simulink model "ANS_GFM_short_term"  (R2021b)
settings: Solver=FixedStepAuto  StartTime=0.0  StopTime=5  FixedStep=Ts  MaxStep=1e-5  RelTol=1e-3
values from neighbouring files (symbols this model uses):
  angle_load = angle(LF.bus(ind_l).Vbus)*180/pi    [init_ANS_GFM_long_term.m]    (also in init_ANS_GFM_short_term.m)
  angleV_LF = Vangle_init/180*pi    [init_ANS_GFM_long_term.m]    (also in init_ANS_GFM_short_term.m)
  awu = 1    [init_ANS_GFM_long_term.m]    (also in init_ANS_GFM_short_term.m)
  C_dc = 1/(Xcdc_pu_or*Zbase_dc_new*100*pi)    [init_ANS_GFM_long_term.m]    (also in init_ANS_GFM_short_term.m)
  C_f = 1/(Xcf_pu_or*Zbase_new*100*pi)    (= 0.013712)    [init_ANS_GFM_long_term.m]    (also in init_ANS_GFM_short_term.m = 0.0141333333333)
  control = 3    [init_ANS_GFM_long_term.m]    (also in init_ANS_GFM_short_term.m = 1)
  D_p = (1/(m_p*w_b))    (= 5209935.26289)    [init_ANS_GFM_long_term.m]    (also in init_ANS_GFM_short_term.m = 5370022.73304)
  Egrid_tmp = 1.054080675694902*400e3    (= 421632.270278)    [init_ANS_GFM_long_term.m]    (also in init_ANS_GFM_short_term.m)
  epsi = 1e-4    (= 0.0001)    [init_ANS_GFM_long_term.m]    (also in init_ANS_GFM_short_term.m)
  eta = m_p*V_m^2    [init_ANS_GFM_long_term.m]    (also in init_ANS_GFM_short_term.m)
  gamma = 2.3    [init_ANS_GFM_long_term.m]    (also in init_ANS_GFM_short_term.m)
  I0_init = [I0_init_a, I0_init_b, I0_init_c]    [init_ANS_GFM_long_term.m]    (also in init_ANS_GFM_short_term.m)
  I_bc = S_bc / (V_bc*sqrt(3))    [init_ANS_GFM_long_term.m]    (also in init_ANS_GFM_short_term.m)
  I_d_int_init = (U_d_int + I_q_int*L_f*w_b - V_d_int - I_d_int*R_f*0)    [init_ANS_GFM_long_term.m]    (also in init_ANS_GFM_short_term.m)
  I_init = [I_init_a, I_init_b, I_init_c]    [init_ANS_GFM_long_term.m]    (also in init_ANS_GFM_short_term.m)
  i_ll = -1.15*(S_bc/Vdc_n)-i_loss_dc    [init_ANS_GFM_long_term.m]    (also in init_ANS_GFM_short_term.m)
  I_max_sat_pu = 1.0 * I_bc *sqrt(2)    [init_ANS_GFM_long_term.m]    (also in init_ANS_GFM_short_term.m)
  I_q_int_init = (U_q_int - I_d_int*L_f*w_b - V_q_int - I_q_int*R_f*0)    [init_ANS_GFM_long_term.m]    (also in init_ANS_GFM_short_term.m)
  i_ul = 1.15*(S_bc/Vdc_n)+i_loss_dc    [init_ANS_GFM_long_term.m]    (also in init_ANS_GFM_short_term.m)
  idppu = 0.95    [init_ANS_GFM_long_term.m]    (also in init_ANS_GFM_short_term.m = 0.92)
  init_dP = -inv(A_pm)*B_pm*dP    [init_ANS_GFM_long_term.m]    (also in init_ANS_GFM_short_term.m)
  init_pm = -inv(A_pm)*B_pm*P_aft    [init_ANS_GFM_long_term.m]    (also in init_ANS_GFM_short_term.m)
  init_tau = -inv(A_tau)*B_tau*idc    [init_ANS_GFM_long_term.m]    (also in init_ANS_GFM_short_term.m)
  J = D_p*tau_f    (= 104198.705258)    [init_ANS_GFM_long_term.m]    (also in init_ANS_GFM_short_term.m = 107400.454661)
  k_dc = eta_1/(Vdc_n*m_p)    [init_ANS_GFM_long_term.m]    (also in init_ANS_GFM_short_term.m)
  K_p = (1/Vdc_n)    [init_ANS_GFM_long_term.m]    (also in init_ANS_GFM_short_term.m)
  K_r = 1/R_dc    [init_ANS_GFM_long_term.m]    (also in init_ANS_GFM_short_term.m)
  Kff_i = 1    [init_ANS_GFM_long_term.m]    (also in init_ANS_GFM_short_term.m)
  Kff_v = 1    [init_ANS_GFM_long_term.m]    (also in init_ANS_GFM_short_term.m)
  Ki_i = (1/n)*1.19    (= 0.0520711785298)    [init_ANS_GFM_long_term.m]    (also in init_ANS_GFM_short_term.m = 0.0505188679245)
  Ki_pll = 4255.3    [init_ANS_GFM_long_term.m]    (also in init_ANS_GFM_short_term.m)
  Ki_v = (n)*1.161022    (= 26.5332227733)    [init_ANS_GFM_long_term.m]    (also in init_ANS_GFM_short_term.m = 27.3485182222)
  ki_v_ac = 2*0.25    (= 0.5)    [init_ANS_GFM_long_term.m]    (also in init_ANS_GFM_short_term.m)
  Kp_i = 0.738891/n    (= 0.032331869895)    [init_ANS_GFM_long_term.m]    (also in init_ANS_GFM_short_term.m = 0.0313680141509)
  Kp_pll = 92    [init_ANS_GFM_long_term.m]    (also in init_ANS_GFM_short_term.m)
  Kp_v = 0.52*n    (= 11.8837333333)    [init_ANS_GFM_long_term.m]    (also in init_ANS_GFM_short_term.m = 12.2488888889)
  kp_v_ac = 0.001    [init_ANS_GFM_long_term.m]    (also in init_ANS_GFM_short_term.m)
  Kpl = 5.0    (= 5)    [init_ANS_GFM_long_term.m]    (also in init_ANS_GFM_short_term.m)
  L1 = cf/sqrt(1+RX^2)*(400e3)^2/Skss/(100*pi)    [init_ANS_GFM_long_term.m]    (also in init_ANS_GFM_short_term.m)
  L_f = Xlf_pu_or*Zbase_new/100/pi    (= 4.37572928821e-06)    [init_ANS_GFM_long_term.m]    (also in init_ANS_GFM_short_term.m = 4.24528301887e-06)
  Lf = 1e6/100/pi    (= 3183.09886184)    [init_ANS_GFM_long_term.m]    (also in init_ANS_GFM_short_term.m = 0.0636619772368)
  m_p = (2*pi*0.5)/(S_bc)    (= 6.10967066042e-10)    [init_ANS_GFM_long_term.m]    (also in init_ANS_GFM_short_term.m = 5.92753330866e-10)
  n = 1/Zb    (= 22.8533333333)    [init_ANS_GFM_long_term.m]    (also in init_ANS_GFM_short_term.m = 23.5555555556)
  P_LF_si = P_LF*S_b    [init_ANS_GFM_long_term.m]    (also in init_ANS_GFM_short_term.m)
  ps = 4440e6/S_bc    (= 0.863477246208)    [init_ANS_GFM_long_term.m]    (also in init_ANS_GFM_short_term.m = 0.837735849057)
  Q_LF_si = Q_LF*S_b    [init_ANS_GFM_long_term.m]    (also in init_ANS_GFM_short_term.m)
  qs = Q_LF*S_b/S_bc    [init_ANS_GFM_long_term.m]    (also in init_ANS_GFM_short_term.m)
  R1 = RX*cf/sqrt(1+RX^2)*(400e3)^2/Skss    [init_ANS_GFM_long_term.m]    (also in init_ANS_GFM_short_term.m)
  R_dc = Rdc_pu_or*Zbase_dc_new    [init_ANS_GFM_long_term.m]    (also in init_ANS_GFM_short_term.m)
  R_f = Rf_pu_or*Zbase_new    (= 2.18786464411e-05)    [init_ANS_GFM_long_term.m]    (also in init_ANS_GFM_short_term.m = 2.12264150943e-05)
  Rf = 1e6    (= 1000000)    [init_ANS_GFM_long_term.m]    (also in init_ANS_GFM_short_term.m = 20)
  S_bc = 5142e6    (= 5142000000)    [init_ANS_GFM_long_term.m]    (also in init_ANS_GFM_short_term.m = 5300000000)
  sat_select = 3    [init_ANS_GFM_long_term.m]    (also in init_ANS_GFM_short_term.m)
  SECM = 3    [init_ANS_GFM_long_term.m]    (also in init_ANS_GFM_short_term.m = 1)
  share_i_load = 1.0    (= 1)    [init_ANS_GFM_long_term.m]    (also in init_ANS_GFM_short_term.m)
  T_en = -0.5    [init_ANS_GFM_long_term.m]    (also in init_ANS_GFM_short_term.m)
  T_off = T_on + 0.1    (= 0.2)    [init_ANS_GFM_long_term.m]    (also in init_ANS_GFM_short_term.m)
  T_on = 0.1    [init_ANS_GFM_long_term.m]    (also in init_ANS_GFM_short_term.m)
  Ts = 2e-6    (= 2e-06)    [init_ANS_GFM_long_term.m]    (also in init_ANS_GFM_short_term.m = 1e-06)
  U_init = [Umag_init_a, Umag_init_b, Umag_init_c]    [init_ANS_GFM_long_term.m]    (also in init_ANS_GFM_short_term.m)
  Uangle_init = angle(V_LF_VSC)*180/pi    [init_ANS_GFM_long_term.m]    (also in init_ANS_GFM_short_term.m)
  Umag_init = abs(V_LF_VSC)*V_bc*sqrt(2/3)    [init_ANS_GFM_long_term.m]    (also in init_ANS_GFM_short_term.m)
  V1_rms = 15e3    (= 15000)    [init_ANS_GFM_long_term.m]    (also in init_ANS_GFM_short_term.m)
  V_d_int = abs(V_LF)*V_bc*sqrt(2/3)    [init_ANS_GFM_long_term.m]    (also in init_ANS_GFM_short_term.m)
  V_d_int_init = (I_d_int + V_q_int*C_f*w_b - I0_d_int)    [init_ANS_GFM_long_term.m]    (also in init_ANS_GFM_short_term.m)
  V_init = [V_init_a, V_init_b, V_init_c]    [init_ANS_GFM_long_term.m]    (also in init_ANS_GFM_short_term.m)
  V_m = sqrt(2/3)*V_bc    [init_ANS_GFM_long_term.m]    (also in init_ANS_GFM_short_term.m)
  V_q_int_init = (I_q_int - V_d_int*C_f*w_b - I0_q_int)    [init_ANS_GFM_long_term.m]    (also in init_ANS_GFM_short_term.m)
  Vdc_n = 3*V_m    [init_ANS_GFM_long_term.m]    (also in init_ANS_GFM_short_term.m)
  Vref = V_LF_mag*V_m    [init_ANS_GFM_long_term.m]    (also in init_ANS_GFM_short_term.m)
  w_b = 2*pi*f_b    (= 314.159265359)    [init_ANS_GFM_long_term.m]    (also in init_ANS_GFM_short_term.m)
  w_f = 2*pi*5    (= 31.4159265359)    [init_ANS_GFM_long_term.m]    (also in init_ANS_GFM_short_term.m)
  Zbase_new = V1_rms^2/S_bc    (= 0.0437572928821)    [init_ANS_GFM_long_term.m]    (also in init_ANS_GFM_short_term.m = 0.0424528301887)
undefined symbols (not defined in the file or in its folder): A_pm, A_tau, B_pm, B_tau, C_pm, C_tau, D_pm, D_tau, find_system, idq0_init, Pm, sm_init, v_d, v_q, Ve
libraries: spsBreakerLib x270, spsGroundLib x21, spsThreePhaseSeriesRLCBranchLib x12, spsabctodq0Lib x11, simulink x9, spsEdgeDetectorLib x8, spsThreePhaseVIMeasurementLib x7, spsLoadFlowBusLib x7, spsSeriesRLCBranchLib x6, spsControlledVoltageSourceLib x6, spsCurrentMeasurementLib x6, spsVoltageMeasurementLib x6
(part 7 of 7)

== system ANS_GFM_short_term/OLTC/ OLTC Control/Set Reset ==
  Tap : Inport
  Hit Crossing : HitCross  HitCrossingOffset=0.5  HitCrossingDirection=rising
  Hit Crossing1 : HitCross  HitCrossingOffset=-0.5  HitCrossingDirection=falling
  Set : Outport  VectorParamsAs1DForOutWhenUnconnected=off
  Reset : Outport  Port=2  VectorParamsAs1DForOutWhenUnconnected=off
  wires:
  Hit Crossing/1 -> Set/1
  Tap/1 -> Hit Crossing1/1, Hit Crossing/1
  Hit Crossing1/1 -> Reset/1

== system ANS_GFM_short_term/OLTC/ OLTC Control/Tap Changer Control ==
  Up : Inport
  Down : Inport  Port=2
  Constant : Constant  Value=-1
  Constant1 : Constant
  Determine tap position : Subsystem  TreatAsAtomicUnit=on
  Edge Detector1 : spsEdgeDetectorLib/Edge Detector  model=Rising  ic=0  Ts=0
      settings: SourceProductBaseCode=PS
  Logical Operator : Logic  Operator=OR  AllPortsSameDT=off
  Logical Operator1 : Logic  AllPortsSameDT=off
  Mechanical Delay : TransportDelay  DelayTime=MecDelay  InitialOutput=InitialPosition
  Memory : Memory  InitialCondition=1  InheritSampleTime=on
  Relational Operator : RelationalOperator  Operator===  OutDataTypeStr=float('double')  RndMeth=Nearest
  Switch : Switch  Threshold=0.5  SaturateOnIntegerOverflow=on
  TapNo : Outport  VectorParamsAs1DForOutWhenUnconnected=off
  Ready : Outport  Port=2  VectorParamsAs1DForOutWhenUnconnected=off
  wires:
  Mechanical Delay/1 -> TapNo/1, Relational Operator/2
  Logical Operator1/1 -> Determine tap position/Trigger
  Up/1 -> Logical Operator/1
  Down/1 -> Logical Operator/2, Switch/2
  Constant/1 -> Switch/1
  Constant1/1 -> Switch/3
  Switch/1 -> Determine tap position/1(NewTap)
  Determine tap position/1(TapNo) -> Mechanical Delay/1, Relational Operator/1
  Relational Operator/1 -> Memory/1
  Memory/1 -> Logical Operator1/1, Ready/1
  Logical Operator/1 -> Edge Detector1/1
  Edge Detector1/1 -> Logical Operator1/2

== system ANS_GFM_short_term/OLTC/OLTCA/Tapped Winding Inversion ==
  Inv : Inport
  Logical Operator : Logic  Operator=NOT  AllPortsSameDT=off
  SwInv1 : spsBreakerLib/Breaker  InitialState=InitialStateInv1  SwitchingTimes="[ 1/60  5/60 ]"  External=on  BreakerResistance=Rswitch  SnubberResistance=1e8  SnubberCapacitance=inf  Measurements=None  MoreParameters=off  NoBreakLoop=off
      settings: SourceProductBaseCode=PS
  SwInv2 : spsBreakerLib/Breaker  InitialState=InitialStateInv2  SwitchingTimes="[ 1/60  5/60 ]"  External=on  BreakerResistance=Rswitch  SnubberResistance=1e8  SnubberCapacitance=inf  Measurements=None  MoreParameters=off  NoBreakLoop=off
      settings: SourceProductBaseCode=PS
  SwInv3 : spsBreakerLib/Breaker  InitialState=InitialStateInv3  SwitchingTimes="[ 1/60  5/60 ]"  External=on  BreakerResistance=Rswitch  SnubberResistance=1e8  SnubberCapacitance=inf  Measurements=None  MoreParameters=off  NoBreakLoop=off
      settings: SourceProductBaseCode=PS
  SwInv4 : spsBreakerLib/Breaker  InitialState=InitialStateInv4  SwitchingTimes="[ 1/60  5/60 ]"  External=on  BreakerResistance=Rswitch  SnubberResistance=1e8  SnubberCapacitance=inf  Measurements=None  MoreParameters=off  NoBreakLoop=off
      settings: SourceProductBaseCode=PS
  In1 : PMIOPort  Side=Left
  In2 : PMIOPort  Port=2  Side=Left
  Out1 : PMIOPort  Port=3  Side=Right
  Out2 : PMIOPort  Port=4  Side=Right
  wires:
  Logical Operator/1 -> SwInv4/1, SwInv2/1
  Inv/1 -> Logical Operator/1, SwInv3/1, SwInv1/1
  connections:
  SwInv4/LConn1 -- SwInv3/LConn1 -- In2/RConn1
  Out2/RConn1 -- SwInv2/RConn1 -- SwInv3/RConn1
  SwInv2/LConn1 -- SwInv1/LConn1 -- In1/RConn1
  Out1/RConn1 -- SwInv4/RConn1 -- SwInv1/RConn1

== system ANS_GFM_short_term/OLTC/OLTCA1/Tapped Winding Inversion ==
  Inv : Inport
  Logical Operator : Logic  Operator=NOT  AllPortsSameDT=off
  SwInv1 : spsBreakerLib/Breaker  InitialState=InitialStateInv1  SwitchingTimes="[ 1/60  5/60 ]"  External=on  BreakerResistance=Rswitch  SnubberResistance=1e8  SnubberCapacitance=inf  Measurements=None  MoreParameters=off  NoBreakLoop=off
      settings: SourceProductBaseCode=PS
  SwInv2 : spsBreakerLib/Breaker  InitialState=InitialStateInv2  SwitchingTimes="[ 1/60  5/60 ]"  External=on  BreakerResistance=Rswitch  SnubberResistance=1e8  SnubberCapacitance=inf  Measurements=None  MoreParameters=off  NoBreakLoop=off
      settings: SourceProductBaseCode=PS
  SwInv3 : spsBreakerLib/Breaker  InitialState=InitialStateInv3  SwitchingTimes="[ 1/60  5/60 ]"  External=on  BreakerResistance=Rswitch  SnubberResistance=1e8  SnubberCapacitance=inf  Measurements=None  MoreParameters=off  NoBreakLoop=off
      settings: SourceProductBaseCode=PS
  SwInv4 : spsBreakerLib/Breaker  InitialState=InitialStateInv4  SwitchingTimes="[ 1/60  5/60 ]"  External=on  BreakerResistance=Rswitch  SnubberResistance=1e8  SnubberCapacitance=inf  Measurements=None  MoreParameters=off  NoBreakLoop=off
      settings: SourceProductBaseCode=PS
  In1 : PMIOPort  Side=Left
  In2 : PMIOPort  Port=2  Side=Left
  Out1 : PMIOPort  Port=3  Side=Right
  Out2 : PMIOPort  Port=4  Side=Right
  wires:
  Logical Operator/1 -> SwInv4/1, SwInv2/1
  Inv/1 -> Logical Operator/1, SwInv3/1, SwInv1/1
  connections:
  SwInv4/LConn1 -- SwInv3/LConn1 -- In2/RConn1
  Out2/RConn1 -- SwInv2/RConn1 -- SwInv3/RConn1
  SwInv2/LConn1 -- SwInv1/LConn1 -- In1/RConn1
  Out1/RConn1 -- SwInv4/RConn1 -- SwInv1/RConn1

== system ANS_GFM_short_term/OLTC/OLTCA2/Tapped Winding Inversion ==
  Inv : Inport
  Logical Operator : Logic  Operator=NOT  AllPortsSameDT=off
  SwInv1 : spsBreakerLib/Breaker  InitialState=InitialStateInv1  SwitchingTimes="[ 1/60  5/60 ]"  External=on  BreakerResistance=Rswitch  SnubberResistance=1e8  SnubberCapacitance=inf  Measurements=None  MoreParameters=off  NoBreakLoop=off
      settings: SourceProductBaseCode=PS
  SwInv2 : spsBreakerLib/Breaker  InitialState=InitialStateInv2  SwitchingTimes="[ 1/60  5/60 ]"  External=on  BreakerResistance=Rswitch  SnubberResistance=1e8  SnubberCapacitance=inf  Measurements=None  MoreParameters=off  NoBreakLoop=off
      settings: SourceProductBaseCode=PS
  SwInv3 : spsBreakerLib/Breaker  InitialState=InitialStateInv3  SwitchingTimes="[ 1/60  5/60 ]"  External=on  BreakerResistance=Rswitch  SnubberResistance=1e8  SnubberCapacitance=inf  Measurements=None  MoreParameters=off  NoBreakLoop=off
      settings: SourceProductBaseCode=PS
  SwInv4 : spsBreakerLib/Breaker  InitialState=InitialStateInv4  SwitchingTimes="[ 1/60  5/60 ]"  External=on  BreakerResistance=Rswitch  SnubberResistance=1e8  SnubberCapacitance=inf  Measurements=None  MoreParameters=off  NoBreakLoop=off
      settings: SourceProductBaseCode=PS
  In1 : PMIOPort  Side=Left
  In2 : PMIOPort  Port=2  Side=Left
  Out1 : PMIOPort  Port=3  Side=Right
  Out2 : PMIOPort  Port=4  Side=Right
  wires:
  Logical Operator/1 -> SwInv4/1, SwInv2/1
  Inv/1 -> Logical Operator/1, SwInv3/1, SwInv1/1
  connections:
  SwInv4/LConn1 -- SwInv3/LConn1 -- In2/RConn1
  Out2/RConn1 -- SwInv2/RConn1 -- SwInv3/RConn1
  SwInv2/LConn1 -- SwInv1/LConn1 -- In1/RConn1
  Out1/RConn1 -- SwInv4/RConn1 -- SwInv1/RConn1

== system ANS_GFM_short_term/OLTC/OLTCA3/Tapped Winding Inversion ==
  Inv : Inport
  Logical Operator : Logic  Operator=NOT  AllPortsSameDT=off
  SwInv1 : spsBreakerLib/Breaker  InitialState=InitialStateInv1  SwitchingTimes="[ 1/60  5/60 ]"  External=on  BreakerResistance=1e-8  SnubberResistance=1e8  SnubberCapacitance=inf  Measurements=None  MoreParameters=off  NoBreakLoop=off
      settings: SourceProductBaseCode=PS
  SwInv2 : spsBreakerLib/Breaker  InitialState=InitialStateInv2  SwitchingTimes="[ 1/60  5/60 ]"  External=on  BreakerResistance=1e-8  SnubberResistance=1e8  SnubberCapacitance=inf  Measurements=None  MoreParameters=off  NoBreakLoop=off
      settings: SourceProductBaseCode=PS
  SwInv3 : spsBreakerLib/Breaker  InitialState=InitialStateInv3  SwitchingTimes="[ 1/60  5/60 ]"  External=on  BreakerResistance=1e-8  SnubberResistance=1e8  SnubberCapacitance=inf  Measurements=None  MoreParameters=off  NoBreakLoop=off
      settings: SourceProductBaseCode=PS
  SwInv4 : spsBreakerLib/Breaker  InitialState=InitialStateInv4  SwitchingTimes="[ 1/60  5/60 ]"  External=on  BreakerResistance=1e-8  SnubberResistance=1e8  SnubberCapacitance=inf  Measurements=None  MoreParameters=off  NoBreakLoop=off
      settings: SourceProductBaseCode=PS
  In1 : PMIOPort  Side=Left
  In2 : PMIOPort  Port=2  Side=Left
  Out1 : PMIOPort  Port=3  Side=Right
  Out2 : PMIOPort  Port=4  Side=Right
  wires:
  Logical Operator/1 -> SwInv4/1, SwInv2/1
  Inv/1 -> Logical Operator/1, SwInv3/1, SwInv1/1
  connections:
  SwInv4/LConn1 -- SwInv3/LConn1 -- In2/RConn1
  Out2/RConn1 -- SwInv2/RConn1 -- SwInv3/RConn1
  SwInv2/LConn1 -- SwInv1/LConn1 -- In1/RConn1
  Out1/RConn1 -- SwInv4/RConn1 -- SwInv1/RConn1

== system ANS_GFM_short_term/OLTC/OLTCC1/Tapped Winding Inversion ==
  Inv : Inport
  Logical Operator : Logic  Operator=NOT  AllPortsSameDT=off
  SwInv1 : spsBreakerLib/Breaker  InitialState=InitialStateInv1  SwitchingTimes="[ 1/60  5/60 ]"  External=on  BreakerResistance=1e-6  SnubberResistance=1e8  SnubberCapacitance=inf  Measurements=None  MoreParameters=off  NoBreakLoop=off
      settings: SourceProductBaseCode=PS
  SwInv2 : spsBreakerLib/Breaker  InitialState=InitialStateInv2  SwitchingTimes="[ 1/60  5/60 ]"  External=on  BreakerResistance=1e-6  SnubberResistance=1e8  SnubberCapacitance=inf  Measurements=None  MoreParameters=off  NoBreakLoop=off
      settings: SourceProductBaseCode=PS
  SwInv3 : spsBreakerLib/Breaker  InitialState=InitialStateInv3  SwitchingTimes="[ 1/60  5/60 ]"  External=on  BreakerResistance=1e-6  SnubberResistance=1e8  SnubberCapacitance=inf  Measurements=None  MoreParameters=off  NoBreakLoop=off
      settings: SourceProductBaseCode=PS
  SwInv4 : spsBreakerLib/Breaker  InitialState=InitialStateInv4  SwitchingTimes="[ 1/60  5/60 ]"  External=on  BreakerResistance=1e-6  SnubberResistance=1e8  SnubberCapacitance=inf  Measurements=None  MoreParameters=off  NoBreakLoop=off
      settings: SourceProductBaseCode=PS
  In1 : PMIOPort  Side=Left
  In2 : PMIOPort  Port=2  Side=Left
  Out1 : PMIOPort  Port=3  Side=Right
  Out2 : PMIOPort  Port=4  Side=Right
  wires:
  Logical Operator/1 -> SwInv4/1, SwInv2/1
  Inv/1 -> Logical Operator/1, SwInv3/1, SwInv1/1
  connections:
  SwInv4/LConn1 -- SwInv3/LConn1 -- In2/RConn1
  Out2/RConn1 -- SwInv2/RConn1 -- SwInv3/RConn1
  SwInv2/LConn1 -- SwInv1/LConn1 -- In1/RConn1
  Out1/RConn1 -- SwInv4/RConn1 -- SwInv1/RConn1

== system ANS_GFM_short_term/OLTC/Voltage regulator/MyDelay1 ==
  in : Inport
  AND1 : Logic  IconShape=distinctive  AllPortsSameDT=off  OutDataTypeStr=boolean
  Constant5 : Constant
  Constant7 : Constant  Value=-RegulatorDelay
  Constant8 : Constant  Value=0
  Delay : Delay  Commented=through  DelayLength=1
  Delay1 : Delay  DelayLength=1
  Edge Detector1 : spsEdgeDetectorLib/Edge Detector  model=Rising  ic=0  Ts=0
      settings: SourceProductBaseCode=PS
  Integrator1 : Integrator  ExternalReset=falling  InitialConditionSource=external  InitialCondition=-5
  NOT1 : Logic  Operator=NOT  IconShape=distinctive  AllPortsSameDT=off  OutDataTypeStr=boolean
  Switch2 : Switch
  Switch3 : Switch  Criteria=u2 > Threshold
  out : Outport
  wires:
  Constant5/1 -> Switch2/1, Switch3/1
  Integrator1/1 -> Switch2/2
  Edge Detector1/1 -> NOT1/1
  AND1/1 -> Integrator1/2
  Switch3/1 -> Integrator1/1
  Constant8/1 -> Switch3/3, Switch2/3
  NOT1/1 -> AND1/2
  Constant7/1 -> Integrator1/3
  in/1 -> Delay/1
  Switch2/1 -> out/1, Delay1/1
  Delay/1 -> Switch3/2, AND1/1
  Delay1/1 -> Edge Detector1/1

== system ANS_GFM_short_term/OLTC/Voltage regulator/MyDelay2 ==
  in : Inport
  AND1 : Logic  IconShape=distinctive  AllPortsSameDT=off  OutDataTypeStr=boolean
  Constant5 : Constant
  Constant7 : Constant  Value=-RegulatorDelay
  Constant8 : Constant  Value=0
  Delay : Delay  Commented=through  DelayLength=1
  Delay1 : Delay  DelayLength=1
  Edge Detector1 : spsEdgeDetectorLib/Edge Detector  model=Rising  ic=0  Ts=0
      settings: SourceProductBaseCode=PS
  Integrator1 : Integrator  ExternalReset=falling  InitialConditionSource=external  InitialCondition=-5
  NOT1 : Logic  Operator=NOT  IconShape=distinctive  AllPortsSameDT=off  OutDataTypeStr=boolean
  Switch2 : Switch
  Switch3 : Switch  Criteria=u2 > Threshold
  out : Outport
  wires:
  Constant5/1 -> Switch2/1, Switch3/1
  Integrator1/1 -> Switch2/2
  Edge Detector1/1 -> NOT1/1
  AND1/1 -> Integrator1/2
  Switch3/1 -> Integrator1/1
  Constant8/1 -> Switch3/3, Switch2/3
  NOT1/1 -> AND1/2
  Constant7/1 -> Integrator1/3
  in/1 -> Delay/1
  Switch2/1 -> out/1, Delay1/1
  Delay/1 -> Switch3/2, AND1/1
  Delay1/1 -> Edge Detector1/1

== system ANS_GFM_short_term/OLTC for load flow/ OLTC Control/Set Reset ==
  Tap : Inport
  Hit Crossing : HitCross  HitCrossingOffset=0.5  HitCrossingDirection=rising
  Hit Crossing1 : HitCross  HitCrossingOffset=-0.5  HitCrossingDirection=falling
  Set : Outport  VectorParamsAs1DForOutWhenUnconnected=off
  Reset : Outport  Port=2  VectorParamsAs1DForOutWhenUnconnected=off
  wires:
  Hit Crossing/1 -> Set/1
  Tap/1 -> Hit Crossing1/1, Hit Crossing/1
  Hit Crossing1/1 -> Reset/1

== system ANS_GFM_short_term/OLTC for load flow/ OLTC Control/Tap Changer Control ==
  Up : Inport
  Down : Inport  Port=2
  Constant : Constant  Value=-1
  Constant1 : Constant
  Determine tap position : Subsystem  TreatAsAtomicUnit=on
  Edge Detector1 : spsEdgeDetectorLib/Edge Detector  model=Rising  ic=0  Ts=0
      settings: SourceProductBaseCode=PS
  Logical Operator : Logic  Operator=OR  AllPortsSameDT=off
  Logical Operator1 : Logic  AllPortsSameDT=off
  Mechanical Delay : TransportDelay  DelayTime=MecDelay  InitialOutput=InitialPosition
  Memory : Memory  InitialCondition=1  InheritSampleTime=on
  Relational Operator : RelationalOperator  Operator===  OutDataTypeStr=float('double')  RndMeth=Nearest
  Switch : Switch  Threshold=0.5  SaturateOnIntegerOverflow=on
  TapNo : Outport  VectorParamsAs1DForOutWhenUnconnected=off
  Ready : Outport  Port=2  VectorParamsAs1DForOutWhenUnconnected=off
  wires:
  Mechanical Delay/1 -> TapNo/1, Relational Operator/2
  Logical Operator1/1 -> Determine tap position/Trigger
  Up/1 -> Logical Operator/1
  Down/1 -> Logical Operator/2, Switch/2
  Constant/1 -> Switch/1
  Constant1/1 -> Switch/3
  Switch/1 -> Determine tap position/1(NewTap)
  Determine tap position/1(TapNo) -> Mechanical Delay/1, Relational Operator/1
  Relational Operator/1 -> Memory/1
  Memory/1 -> Logical Operator1/1, Ready/1
  Logical Operator/1 -> Edge Detector1/1
  Edge Detector1/1 -> Logical Operator1/2

== system ANS_GFM_short_term/OLTC for load flow/OLTCA/Tapped Winding Inversion ==
  Inv : Inport
  Logical Operator : Logic  Operator=NOT  AllPortsSameDT=off
  SwInv1 : spsBreakerLib/Breaker  InitialState=InitialStateInv1  SwitchingTimes="[ 1/60  5/60 ]"  External=on  BreakerResistance=Rswitch  SnubberResistance=1e8  SnubberCapacitance=inf  Measurements=None  MoreParameters=off  NoBreakLoop=off
      settings: SourceProductBaseCode=PS
  SwInv2 : spsBreakerLib/Breaker  InitialState=InitialStateInv2  SwitchingTimes="[ 1/60  5/60 ]"  External=on  BreakerResistance=Rswitch  SnubberResistance=1e8  SnubberCapacitance=inf  Measurements=None  MoreParameters=off  NoBreakLoop=off
      settings: SourceProductBaseCode=PS
  SwInv3 : spsBreakerLib/Breaker  InitialState=InitialStateInv3  SwitchingTimes="[ 1/60  5/60 ]"  External=on  BreakerResistance=Rswitch  SnubberResistance=1e8  SnubberCapacitance=inf  Measurements=None  MoreParameters=off  NoBreakLoop=off
      settings: SourceProductBaseCode=PS
  SwInv4 : spsBreakerLib/Breaker  InitialState=InitialStateInv4  SwitchingTimes="[ 1/60  5/60 ]"  External=on  BreakerResistance=Rswitch  SnubberResistance=1e8  SnubberCapacitance=inf  Measurements=None  MoreParameters=off  NoBreakLoop=off
      settings: SourceProductBaseCode=PS
  In1 : PMIOPort  Side=Left
  In2 : PMIOPort  Port=2  Side=Left
  Out1 : PMIOPort  Port=3  Side=Right
  Out2 : PMIOPort  Port=4  Side=Right
  wires:
  Logical Operator/1 -> SwInv4/1, SwInv2/1
  Inv/1 -> Logical Operator/1, SwInv3/1, SwInv1/1
  connections:
  SwInv4/LConn1 -- SwInv3/LConn1 -- In2/RConn1
  Out2/RConn1 -- SwInv2/RConn1 -- SwInv3/RConn1
  SwInv2/LConn1 -- SwInv1/LConn1 -- In1/RConn1
  Out1/RConn1 -- SwInv4/RConn1 -- SwInv1/RConn1

== system ANS_GFM_short_term/OLTC for load flow/OLTCA1/Tapped Winding Inversion ==
  Inv : Inport
  Logical Operator : Logic  Operator=NOT  AllPortsSameDT=off
  SwInv1 : spsBreakerLib/Breaker  InitialState=InitialStateInv1  SwitchingTimes="[ 1/60  5/60 ]"  External=on  BreakerResistance=Rswitch  SnubberResistance=1e8  SnubberCapacitance=inf  Measurements=None  MoreParameters=off  NoBreakLoop=off
      settings: SourceProductBaseCode=PS
  SwInv2 : spsBreakerLib/Breaker  InitialState=InitialStateInv2  SwitchingTimes="[ 1/60  5/60 ]"  External=on  BreakerResistance=Rswitch  SnubberResistance=1e8  SnubberCapacitance=inf  Measurements=None  MoreParameters=off  NoBreakLoop=off
      settings: SourceProductBaseCode=PS
  SwInv3 : spsBreakerLib/Breaker  InitialState=InitialStateInv3  SwitchingTimes="[ 1/60  5/60 ]"  External=on  BreakerResistance=Rswitch  SnubberResistance=1e8  SnubberCapacitance=inf  Measurements=None  MoreParameters=off  NoBreakLoop=off
      settings: SourceProductBaseCode=PS
  SwInv4 : spsBreakerLib/Breaker  InitialState=InitialStateInv4  SwitchingTimes="[ 1/60  5/60 ]"  External=on  BreakerResistance=Rswitch  SnubberResistance=1e8  SnubberCapacitance=inf  Measurements=None  MoreParameters=off  NoBreakLoop=off
      settings: SourceProductBaseCode=PS
  In1 : PMIOPort  Side=Left
  In2 : PMIOPort  Port=2  Side=Left
  Out1 : PMIOPort  Port=3  Side=Right
  Out2 : PMIOPort  Port=4  Side=Right
  wires:
  Logical Operator/1 -> SwInv4/1, SwInv2/1
  Inv/1 -> Logical Operator/1, SwInv3/1, SwInv1/1
  connections:
  SwInv4/LConn1 -- SwInv3/LConn1 -- In2/RConn1
  Out2/RConn1 -- SwInv2/RConn1 -- SwInv3/RConn1
  SwInv2/LConn1 -- SwInv1/LConn1 -- In1/RConn1
  Out1/RConn1 -- SwInv4/RConn1 -- SwInv1/RConn1

== system ANS_GFM_short_term/OLTC for load flow/OLTCA2/Tapped Winding Inversion ==
  Inv : Inport
  Logical Operator : Logic  Operator=NOT  AllPortsSameDT=off
  SwInv1 : spsBreakerLib/Breaker  InitialState=InitialStateInv1  SwitchingTimes="[ 1/60  5/60 ]"  External=on  BreakerResistance=Rswitch  SnubberResistance=1e8  SnubberCapacitance=inf  Measurements=None  MoreParameters=off  NoBreakLoop=off
      settings: SourceProductBaseCode=PS
  SwInv2 : spsBreakerLib/Breaker  InitialState=InitialStateInv2  SwitchingTimes="[ 1/60  5/60 ]"  External=on  BreakerResistance=Rswitch  SnubberResistance=1e8  SnubberCapacitance=inf  Measurements=None  MoreParameters=off  NoBreakLoop=off
      settings: SourceProductBaseCode=PS
  SwInv3 : spsBreakerLib/Breaker  InitialState=InitialStateInv3  SwitchingTimes="[ 1/60  5/60 ]"  External=on  BreakerResistance=Rswitch  SnubberResistance=1e8  SnubberCapacitance=inf  Measurements=None  MoreParameters=off  NoBreakLoop=off
      settings: SourceProductBaseCode=PS
  SwInv4 : spsBreakerLib/Breaker  InitialState=InitialStateInv4  SwitchingTimes="[ 1/60  5/60 ]"  External=on  BreakerResistance=Rswitch  SnubberResistance=1e8  SnubberCapacitance=inf  Measurements=None  MoreParameters=off  NoBreakLoop=off
      settings: SourceProductBaseCode=PS
  In1 : PMIOPort  Side=Left
  In2 : PMIOPort  Port=2  Side=Left
  Out1 : PMIOPort  Port=3  Side=Right
  Out2 : PMIOPort  Port=4  Side=Right
  wires:
  Logical Operator/1 -> SwInv4/1, SwInv2/1
  Inv/1 -> Logical Operator/1, SwInv3/1, SwInv1/1
  connections:
  SwInv4/LConn1 -- SwInv3/LConn1 -- In2/RConn1
  Out2/RConn1 -- SwInv2/RConn1 -- SwInv3/RConn1
  SwInv2/LConn1 -- SwInv1/LConn1 -- In1/RConn1
  Out1/RConn1 -- SwInv4/RConn1 -- SwInv1/RConn1

== system ANS_GFM_short_term/OLTC for load flow/OLTCA3/Tapped Winding Inversion ==
  Inv : Inport
  Logical Operator : Logic  Operator=NOT  AllPortsSameDT=off
  SwInv1 : spsBreakerLib/Breaker  InitialState=InitialStateInv1  SwitchingTimes="[ 1/60  5/60 ]"  External=on  BreakerResistance=1e-8  SnubberResistance=1e8  SnubberCapacitance=inf  Measurements=None  MoreParameters=off  NoBreakLoop=off
      settings: SourceProductBaseCode=PS
  SwInv2 : spsBreakerLib/Breaker  InitialState=InitialStateInv2  SwitchingTimes="[ 1/60  5/60 ]"  External=on  BreakerResistance=1e-8  SnubberResistance=1e8  SnubberCapacitance=inf  Measurements=None  MoreParameters=off  NoBreakLoop=off
      settings: SourceProductBaseCode=PS
  SwInv3 : spsBreakerLib/Breaker  InitialState=InitialStateInv3  SwitchingTimes="[ 1/60  5/60 ]"  External=on  BreakerResistance=1e-8  SnubberResistance=1e8  SnubberCapacitance=inf  Measurements=None  MoreParameters=off  NoBreakLoop=off
      settings: SourceProductBaseCode=PS
  SwInv4 : spsBreakerLib/Breaker  InitialState=InitialStateInv4  SwitchingTimes="[ 1/60  5/60 ]"  External=on  BreakerResistance=1e-8  SnubberResistance=1e8  SnubberCapacitance=inf  Measurements=None  MoreParameters=off  NoBreakLoop=off
      settings: SourceProductBaseCode=PS
  In1 : PMIOPort  Side=Left
  In2 : PMIOPort  Port=2  Side=Left
  Out1 : PMIOPort  Port=3  Side=Right
  Out2 : PMIOPort  Port=4  Side=Right
  wires:
  Logical Operator/1 -> SwInv4/1, SwInv2/1
  Inv/1 -> Logical Operator/1, SwInv3/1, SwInv1/1
  connections:
  SwInv4/LConn1 -- SwInv3/LConn1 -- In2/RConn1
  Out2/RConn1 -- SwInv2/RConn1 -- SwInv3/RConn1
  SwInv2/LConn1 -- SwInv1/LConn1 -- In1/RConn1
  Out1/RConn1 -- SwInv4/RConn1 -- SwInv1/RConn1

== system ANS_GFM_short_term/OLTC for load flow/OLTCC1/Tapped Winding Inversion ==
  Inv : Inport
  Logical Operator : Logic  Operator=NOT  AllPortsSameDT=off
  SwInv1 : spsBreakerLib/Breaker  InitialState=InitialStateInv1  SwitchingTimes="[ 1/60  5/60 ]"  External=on  BreakerResistance=1e-6  SnubberResistance=1e8  SnubberCapacitance=inf  Measurements=None  MoreParameters=off  NoBreakLoop=off
      settings: SourceProductBaseCode=PS
  SwInv2 : spsBreakerLib/Breaker  InitialState=InitialStateInv2  SwitchingTimes="[ 1/60  5/60 ]"  External=on  BreakerResistance=1e-6  SnubberResistance=1e8  SnubberCapacitance=inf  Measurements=None  MoreParameters=off  NoBreakLoop=off
      settings: SourceProductBaseCode=PS
  SwInv3 : spsBreakerLib/Breaker  InitialState=InitialStateInv3  SwitchingTimes="[ 1/60  5/60 ]"  External=on  BreakerResistance=1e-6  SnubberResistance=1e8  SnubberCapacitance=inf  Measurements=None  MoreParameters=off  NoBreakLoop=off
      settings: SourceProductBaseCode=PS
  SwInv4 : spsBreakerLib/Breaker  InitialState=InitialStateInv4  SwitchingTimes="[ 1/60  5/60 ]"  External=on  BreakerResistance=1e-6  SnubberResistance=1e8  SnubberCapacitance=inf  Measurements=None  MoreParameters=off  NoBreakLoop=off
      settings: SourceProductBaseCode=PS
  In1 : PMIOPort  Side=Left
  In2 : PMIOPort  Port=2  Side=Left
  Out1 : PMIOPort  Port=3  Side=Right
  Out2 : PMIOPort  Port=4  Side=Right
  wires:
  Logical Operator/1 -> SwInv4/1, SwInv2/1
  Inv/1 -> Logical Operator/1, SwInv3/1, SwInv1/1
  connections:
  SwInv4/LConn1 -- SwInv3/LConn1 -- In2/RConn1
  Out2/RConn1 -- SwInv2/RConn1 -- SwInv3/RConn1
  SwInv2/LConn1 -- SwInv1/LConn1 -- In1/RConn1
  Out1/RConn1 -- SwInv4/RConn1 -- SwInv1/RConn1

== system ANS_GFM_short_term/OLTC for load flow/Voltage regulator/MyDelay1 ==
  in : Inport
  AND1 : Logic  IconShape=distinctive  AllPortsSameDT=off  OutDataTypeStr=boolean
  Constant5 : Constant
  Constant7 : Constant  Value=-RegulatorDelay
  Constant8 : Constant  Value=0
  Delay : Delay  Commented=through  DelayLength=1
  Delay1 : Delay  DelayLength=1
  Edge Detector1 : spsEdgeDetectorLib/Edge Detector  model=Rising  ic=0  Ts=0
      settings: SourceProductBaseCode=PS
  Integrator1 : Integrator  ExternalReset=falling  InitialConditionSource=external  InitialCondition=-5
  NOT1 : Logic  Operator=NOT  IconShape=distinctive  AllPortsSameDT=off  OutDataTypeStr=boolean
  Switch2 : Switch
  Switch3 : Switch  Criteria=u2 > Threshold
  out : Outport
  wires:
  Constant5/1 -> Switch2/1, Switch3/1
  Integrator1/1 -> Switch2/2
  Edge Detector1/1 -> NOT1/1
  AND1/1 -> Integrator1/2
  Switch3/1 -> Integrator1/1
  Constant8/1 -> Switch3/3, Switch2/3
  NOT1/1 -> AND1/2
  Constant7/1 -> Integrator1/3
  in/1 -> Delay/1
  Switch2/1 -> out/1, Delay1/1
  Delay/1 -> Switch3/2, AND1/1
  Delay1/1 -> Edge Detector1/1

== system ANS_GFM_short_term/OLTC for load flow/Voltage regulator/MyDelay2 ==
  in : Inport
  AND1 : Logic  IconShape=distinctive  AllPortsSameDT=off  OutDataTypeStr=boolean
  Constant5 : Constant
  Constant7 : Constant  Value=-RegulatorDelay
  Constant8 : Constant  Value=0
  Delay : Delay  Commented=through  DelayLength=1
  Delay1 : Delay  DelayLength=1
  Edge Detector1 : spsEdgeDetectorLib/Edge Detector  model=Rising  ic=0  Ts=0
      settings: SourceProductBaseCode=PS
  Integrator1 : Integrator  ExternalReset=falling  InitialConditionSource=external  InitialCondition=-5
  NOT1 : Logic  Operator=NOT  IconShape=distinctive  AllPortsSameDT=off  OutDataTypeStr=boolean
  Switch2 : Switch
  Switch3 : Switch  Criteria=u2 > Threshold
  out : Outport
  wires:
  Constant5/1 -> Switch2/1, Switch3/1
  Integrator1/1 -> Switch2/2
  Edge Detector1/1 -> NOT1/1
  AND1/1 -> Integrator1/2
  Switch3/1 -> Integrator1/1
  Constant8/1 -> Switch3/3, Switch2/3
  NOT1/1 -> AND1/2
  Constant7/1 -> Integrator1/3
  in/1 -> Delay/1
  Switch2/1 -> out/1, Delay1/1
  Delay/1 -> Switch3/2, AND1/1
  Delay1/1 -> Edge Detector1/1

== system ANS_GFM_short_term/Synchronous Generator(GENTPJ)/AVR+OEL+PSS/Array logic ==
  u : Inport
  Constant1 : Constant  Value=0
  Constant3 : Constant  Value=-1
  Gain : Gain  Gain=-1
  Switch : Switch
  Switch3 : Switch  Threshold=0.1
  y : Outport  VectorParamsAs1DForOutWhenUnconnected=off
  wires:
  Switch/1 -> Switch3/3
  Constant3/1 -> Switch3/1
  Switch3/1 -> y/1
  u/1 -> Switch/2, Switch/1, Gain/1
  Gain/1 -> Switch3/2
  Constant1/1 -> Switch/3

== system ANS_GFM_short_term/Synchronous Generator(GENTPJ)/AVR+OEL+PSS/DT1-Glied ==
  u : Inport
  Gain4 : Gain  Gain=B
  Gain5 : Gain  Gain=D
  Gain6 : Gain  Gain=C
  Gain7 : Gain  Gain=A
  Integrator : Integrator  InitialCondition=x_init
  Sum3 : Sum  Inputs=|++
  Sum4 : Sum  Inputs=++|
  y : Outport  VectorParamsAs1DForOutWhenUnconnected=off
  wires:
  Gain5/1 -> Sum4/1
  u/1 -> Gain5/1, Gain4/1
  Gain6/1 -> Sum4/2
  Sum3/1 -> Integrator/1
  Gain4/1 -> Sum3/1
  Integrator/1 -> Gain6/1, Gain7/1
  Gain7/1 -> Sum3/2
  Sum4/1 -> y/1

== system ANS_GFM_short_term/Synchronous Generator(GENTPJ)/AVR+OEL+PSS/Lead-Lag ==
  u : Inport
  Gain4 : Gain  Gain=B
  Gain5 : Gain  Gain=D
  Gain6 : Gain  Gain=C
  Gain7 : Gain  Gain=A
  Integrator : Integrator  InitialCondition=x_init
  Sum3 : Sum  Inputs=|++
  Sum4 : Sum  Inputs=++|
  y : Outport  VectorParamsAs1DForOutWhenUnconnected=off
  wires:
  Gain5/1 -> Sum4/1
  u/1 -> Gain5/1, Gain4/1
  Gain6/1 -> Sum4/2
  Sum3/1 -> Integrator/1
  Gain4/1 -> Sum3/1
  Integrator/1 -> Gain6/1, Gain7/1
  Gain7/1 -> Sum3/2
  Sum4/1 -> y/1

== system ANS_GFM_short_term/Synchronous Generator(GENTPJ)/AVR+OEL+PSS/Lead_Lag1 ==
  u : Inport
  Gain4 : Gain  Gain=B
  Gain5 : Gain  Gain=D
  Gain6 : Gain  Gain=C
  Gain7 : Gain  Gain=A
  Integrator : Integrator  InitialCondition=x_init
  Sum3 : Sum  Inputs=|++
  Sum4 : Sum  Inputs=++|
  y : Outport  VectorParamsAs1DForOutWhenUnconnected=off
  wires:
  Gain5/1 -> Sum4/1
  u/1 -> Gain5/1, Gain4/1
  Gain6/1 -> Sum4/2
  Sum3/1 -> Integrator/1
  Gain4/1 -> Sum3/1
  Integrator/1 -> Gain6/1, Gain7/1
  Gain7/1 -> Sum3/2
  Sum4/1 -> y/1

== system ANS_GFM_short_term/Synchronous Generator(GENTPJ)/AVR+OEL+PSS/Lead_Lag2 ==
  u : Inport
  Gain4 : Gain  Gain=B
  Gain5 : Gain  Gain=D
  Gain6 : Gain  Gain=C
  Gain7 : Gain  Gain=A
  Integrator : Integrator  InitialCondition=x_init
  Sum3 : Sum  Inputs=|++
  Sum4 : Sum  Inputs=++|
  y : Outport  VectorParamsAs1DForOutWhenUnconnected=off
  wires:
  Gain5/1 -> Sum4/1
  u/1 -> Gain5/1, Gain4/1
  Gain6/1 -> Sum4/2
  Sum3/1 -> Integrator/1
  Gain4/1 -> Sum3/1
  Integrator/1 -> Gain6/1, Gain7/1
  Gain7/1 -> Sum3/2
  Sum4/1 -> y/1

== system ANS_GFM_short_term/Synchronous Generator(GENTPJ)/Rotor Equations/1+Sd ==
  u : Inport
  El : Inport  Port=2
  Constant : Constant  Value=q
  Constant1 : Constant
  Gain12 : Gain  Gain=S10
  Math Function : Math  Operator=pow  SaturateOnIntegerOverflow=on
  Product : Product
  Sum : Sum  Inputs=|++
  y : Outport
  wires:
  Math Function/1 -> Gain12/1
  Constant/1 -> Math Function/2
  Constant1/1 -> Sum/2
  u/1 -> Product/1
  Gain12/1 -> Sum/1
  El/1 -> Math Function/1
  Sum/1 -> Product/2
  Product/1 -> y/1

== system ANS_GFM_short_term/Synchronous Generator(GENTPJ)/Rotor Equations/1+Sd1 ==
  u : Inport
  El : Inport  Port=2
  Constant : Constant  Value=q
  Constant1 : Constant
  Gain12 : Gain  Gain=S10
  Math Function : Math  Operator=pow  SaturateOnIntegerOverflow=on
  Product : Product
  Sum : Sum  Inputs=|++
  y : Outport
  wires:
  Math Function/1 -> Gain12/1
  Constant/1 -> Math Function/2
  Constant1/1 -> Sum/2
  u/1 -> Product/1
  Gain12/1 -> Sum/1
  El/1 -> Math Function/1
  Sum/1 -> Product/2
  Product/1 -> y/1

== system ANS_GFM_short_term/Synchronous Generator(GENTPJ)/Rotor Equations/1+Sq1 ==
  u : Inport
  El : Inport  Port=2
  Constant : Constant  Value=q
  Constant1 : Constant
  Gain12 : Gain  Gain=S10
  Gain13 : Gain  Gain=Xq/Xd
  Math Function : Math  Operator=pow  SaturateOnIntegerOverflow=on
  Product : Product
  Sum : Sum  Inputs=|++
  y : Outport
  wires:
  Math Function/1 -> Gain12/1
  Constant/1 -> Math Function/2
  Constant1/1 -> Sum/2
  Gain12/1 -> Gain13/1
  u/1 -> Product/1
  Gain13/1 -> Sum/1
  El/1 -> Math Function/1
  Sum/1 -> Product/2
  Product/1 -> y/1

== system ANS_GFM_short_term/Synchronous Generator(GENTPJ)/Rotor Equations/1+Sq2 ==
  u : Inport
  El : Inport  Port=2
  Constant : Constant  Value=q
  Constant1 : Constant
  Gain12 : Gain  Gain=S10
  Gain13 : Gain  Gain=Xq/Xd
  Math Function : Math  Operator=pow  SaturateOnIntegerOverflow=on
  Product : Product
  Sum : Sum  Inputs=|++
  y : Outport
  wires:
  Math Function/1 -> Gain12/1
  Constant/1 -> Math Function/2
  Constant1/1 -> Sum/2
  Gain12/1 -> Gain13/1
  u/1 -> Product/1
  Gain13/1 -> Sum/1
  El/1 -> Math Function/1
  Sum/1 -> Product/2
  Product/1 -> y/1

== system ANS_GFM_short_term/Synchronous Generator(GENTPJ)/Stator Equations/1+Sd ==
  u : Inport
  El : Inport  Port=2
  Constant : Constant  Value=q
  Constant1 : Constant
  Divide : Product  Inputs=*/
  Gain12 : Gain  Gain=S10
  Math Function : Math  Operator=pow  SaturateOnIntegerOverflow=on
  Sum : Sum  Inputs=|++
  y : Outport
  wires:
  Math Function/1 -> Gain12/1
  Constant/1 -> Math Function/2
  Constant1/1 -> Sum/2
  u/1 -> Divide/1
  Gain12/1 -> Sum/1
  El/1 -> Math Function/1
  Sum/1 -> Divide/2
  Divide/1 -> y/1

== system ANS_GFM_short_term/Synchronous Generator(GENTPJ)/Stator Equations/1+Sq ==
  u : Inport
  El : Inport  Port=2
  Constant : Constant  Value=q
  Constant1 : Constant
  Divide : Product  Inputs=*/
  Gain12 : Gain  Gain=S10
  Gain13 : Gain  Gain=Xq/Xd
  Math Function : Math  Operator=pow  SaturateOnIntegerOverflow=on
  Sum : Sum  Inputs=|++
  y : Outport
  wires:
  Math Function/1 -> Gain12/1
  Constant/1 -> Math Function/2
  Constant1/1 -> Sum/2
  Gain12/1 -> Gain13/1
  u/1 -> Divide/1
  Gain13/1 -> Sum/1
  El/1 -> Math Function/1
  Sum/1 -> Divide/2
  Divide/1 -> y/1

== system ANS_GFM_short_term/GFM Converter/GFM controls/dVOC  - kappa=pi//2/APC ==
  p : Inport
  p* : Inport  Port=2
  v : Inport  Port=3
  v* : Inport  Port=4
  Constant1 : Constant  Value=epsi
  Divide : Product  Inputs=*/
  Divide1 : Product  Inputs=*/
  Gain : Gain  Gain=eta
  Gain1 : Gain  Gain=w_f
  Integrator : Integrator  InitialCondition=P_LF_si
  Square : Math  Operator=square  SignedPower=on  SaturateOnIntegerOverflow=on
  Square1 : Math  Operator=square  SignedPower=on  SaturateOnIntegerOverflow=on
  Sum : Sum  Inputs=|++
  Sum1 : Sum  Inputs=|-+
  Sum2 : Sum  Inputs=|+-
  dw : Outport  VectorParamsAs1DForOutWhenUnconnected=off
  wires:
  p*/1 -> Divide1/1
  v/1 -> Square1/1
  Constant1/1 -> Sum/1
  Sum/1 -> Divide/2
  v*/1 -> Square/1
  Square/1 -> Divide1/2
  Square1/1 -> Sum/2
  Divide/1 -> Sum1/1
  Divide1/1 -> Sum1/2
  Sum1/1 -> Gain/1
  Gain/1 -> dw/1
  Integrator/1 -> Divide/1, Sum2/2
  Gain1/1 -> Integrator/1
  Sum2/1 -> Gain1/1
  p/1 -> Sum2/1

== system ANS_GFM_short_term/GFM Converter/GFM controls/dVOC  - kappa=pi//2/P-AVR ==
  v : Inport
  v* : Inport  Port=2
  Divide : Product  Inputs=*/
  Gain : Gain  Gain=1400/10
  Square : Math  Operator=square  SignedPower=on  SaturateOnIntegerOverflow=on
  Square1 : Math  Operator=square  SignedPower=on  SaturateOnIntegerOverflow=on
  Sum1 : Sum  Inputs=|-+
  dv2 : Outport  VectorParamsAs1DForOutWhenUnconnected=off
  wires:
  v/1 -> Square1/1
  v*/1 -> Square/1
  Square/1 -> Sum1/2, Divide/2
  Sum1/1 -> Gain/1
  Square1/1 -> Sum1/1
  Gain/1 -> Divide/1
  Divide/1 -> dv2/1

== system ANS_GFM_short_term/GFM Converter/GFM controls/dVOC  - kappa=pi//2/RPC ==
  q : Inport
  q* : Inport  Port=2
  v : Inport  Port=3
  v* : Inport  Port=4
  Constant : Constant  Value=10
  Divide : Product  Inputs=*/
  Divide1 : Product  Inputs=*/
  Gain : Gain  Gain=eta
  Gain1 : Gain  Gain=w_f
  Integrator : Integrator  InitialCondition=Q_LF_si
  Square : Math  Operator=square  SignedPower=on  SaturateOnIntegerOverflow=on
  Square1 : Math  Operator=square  SignedPower=on  SaturateOnIntegerOverflow=on
  Sum : Sum  Inputs=|++
  Sum1 : Sum  Inputs=|-+
  Sum2 : Sum  Inputs=|+-
  dv1 : Outport  VectorParamsAs1DForOutWhenUnconnected=off
  wires:
  q*/1 -> Divide1/1
  Constant/1 -> Sum/1
  Sum/1 -> Divide/2
  v*/1 -> Square/1
  Square/1 -> Divide1/2
  Square1/1 -> Sum/2
  Divide/1 -> Sum1/1
  Divide1/1 -> Sum1/2
  Sum1/1 -> Gain/1
  Gain/1 -> dv1/1
  v/1 -> Square1/1
  Integrator/1 -> Divide/1, Sum2/2
  Gain1/1 -> Integrator/1
  Sum2/1 -> Gain1/1
  q/1 -> Sum2/1

== system ANS_GFM_short_term/OLTC/ OLTC Control/Tap Changer Control/Determine tap position ==
  NewTap : Inport
  Trigger : TriggerPort  VariantControl=Variant
  Memory : Memory  InitialCondition=InitialPosition  InheritSampleTime=on
  Saturation : Saturate  UpperLimit=MinMaxTap(2)  LowerLimit=MinMaxTap(1)
  Sum : Sum  Inputs=|++  SaturateOnIntegerOverflow=on
  TapNo : Outport  InitialOutput=InitialPosition  VectorParamsAs1DForOutWhenUnconnected=off
  wires:
  NewTap/1 -> Sum/1
  Sum/1 -> Saturation/1
  Memory/1 -> Sum/2
  Saturation/1 -> TapNo/1, Memory/1

== system ANS_GFM_short_term/OLTC for load flow/ OLTC Control/Tap Changer Control/Determine tap position ==
  NewTap : Inport
  Trigger : TriggerPort  VariantControl=Variant
  Memory : Memory  InitialCondition=InitialPosition  InheritSampleTime=on
  Saturation : Saturate  UpperLimit=MinMaxTap(2)  LowerLimit=MinMaxTap(1)
  Sum : Sum  Inputs=|++  SaturateOnIntegerOverflow=on
  TapNo : Outport  InitialOutput=InitialPosition  VectorParamsAs1DForOutWhenUnconnected=off
  wires:
  NewTap/1 -> Sum/1
  Sum/1 -> Saturation/1
  Memory/1 -> Sum/2
  Saturation/1 -> TapNo/1, Memory/1

== matlab function ANS_GFM_short_term/GFM Converter/GFM controls/VSM Control/MATLAB Function1 ==
  data: M_fi_f input; theta input; w input; e output
function e = EMF(M_fi_f, theta, w)
e=w*M_fi_f*[sin(theta) sin(theta-(2*pi/3)) sin(theta-(4*pi/3))]';
end
